simulink model "Cart_Pendulum_9329013"  (R2017b)
settings: Solver=FixedStepAuto  StartTime=0.0  StopTime=10.0  FixedStep=0.05  RelTol=1e-3
values from neighbouring files (symbols this model uses):
  g = 9.81    [CP_ContrSys_Lin_a_Mainfile_n9329013.m]    (also in CP_ContrSys_Lin_b_Mainfile_n9329013.m; MainFile_9329013.m; MainFile_Linearised_a_9329013.m; MainFile_Linearised_b_9329013.m)
  l = 0.2    [CP_ContrSys_Lin_a_Mainfile_n9329013.m]    (also in CP_ContrSys_Lin_b_Mainfile_n9329013.m; MainFile_9329013.m; MainFile_Linearised_a_9329013.m; MainFile_Linearised_b_9329013.m)
  m = 0.15    [CP_ContrSys_Lin_a_Mainfile_n9329013.m]    (also in CP_ContrSys_Lin_b_Mainfile_n9329013.m; MainFile_9329013.m; MainFile_Linearised_a_9329013.m; MainFile_Linearised_b_9329013.m)
  Mc = 0.4    [CP_ContrSys_Lin_a_Mainfile_n9329013.m]    (also in CP_ContrSys_Lin_b_Mainfile_n9329013.m; MainFile_9329013.m; MainFile_Linearised_a_9329013.m; MainFile_Linearised_b_9329013.m)
settings Model: Creator=Koh Kim Hai  LastModifiedBy=Koh Kim Hai

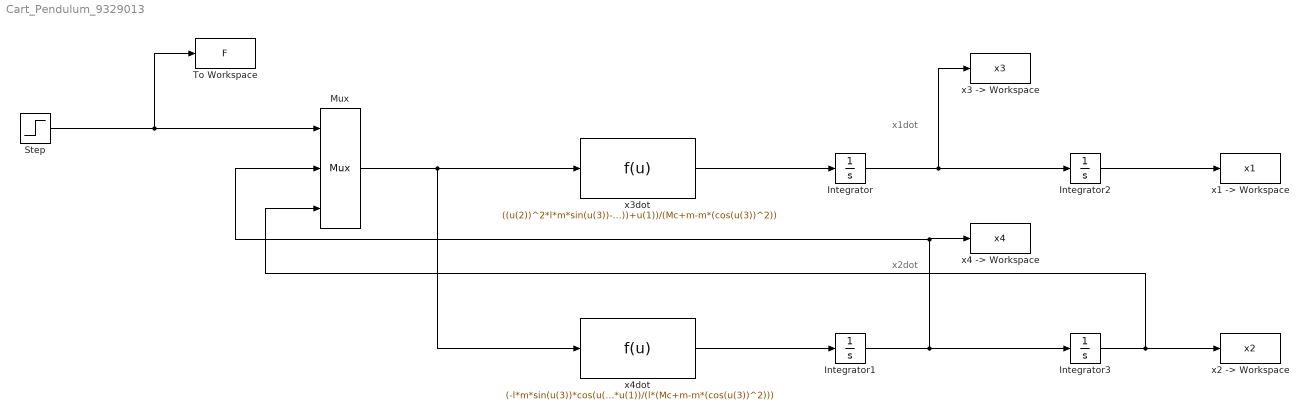
== system Cart_Pendulum_9329013 ==
  note: x2dot
  note: x1dot
  Integrator{,1..3} (4 alike) : Integrator
  Mux : Mux  Inputs=3
  Step : Step  After=0.1  SampleTime=0
  To Workspace : ToWorkspace  VariableName=F  SampleTime=-1
  "x1 -> Workspace" : ToWorkspace  VariableName=x1  SampleTime=-1
  "x2 -> Workspace" : ToWorkspace  VariableName=x2  SampleTime=-1
  "x3 -> Workspace" : ToWorkspace  VariableName=x3  SampleTime=-1
  x3dot : Fcn  Expr=((u(2))^2*l*m*sin(u(3))-g*m*sin(u(3))*cos(u(3))+u(1))/(Mc+m-m*(cos(u(3))^2))
  "x4 -> Workspace" : ToWorkspace  VariableName=x4  SampleTime=-1
  x4dot : Fcn  Expr=(-l*m*sin(u(3))*cos(u(3))*(u(2))^2+g*(Mc+m)*sin(u(3))-cos(u(3))*u(1))/(l*(Mc+m-m*(cos(u(3))^2)))
  wires:
  x3dot/1 -> Integrator/1
  x4dot/1 -> Integrator1/1
  Integrator/1 -> "x3 -> Workspace"/1, Integrator2/1
  Integrator1/1 -> Mux/2, "x4 -> Workspace"/1, Integrator3/1
  Integrator2/1 -> "x1 -> Workspace"/1
  Integrator3/1 -> Mux/3, "x2 -> Workspace"/1
  Step/1 -> To Workspace/1, Mux/1
  Mux/1 -> x4dot/1, x3dot/1
